simulink model "lab"  (Simulink 7.4)
settings: Solver=ode45  StartTime=0.0  StopTime=1  RelTol=1e-6
settings Model: Creator=im42741  LastModifiedBy=ks44349
settings OptimizationCC: InitFltsAndDblsToZero=on
settings DebuggingCC: SaveWithParameterizedLinksMsg=none  SignalResolutionControl=TryResolveAllWithWarning
settings GRTTargetCC: TargetFcnLib=ansi_tfl_tmw.mat

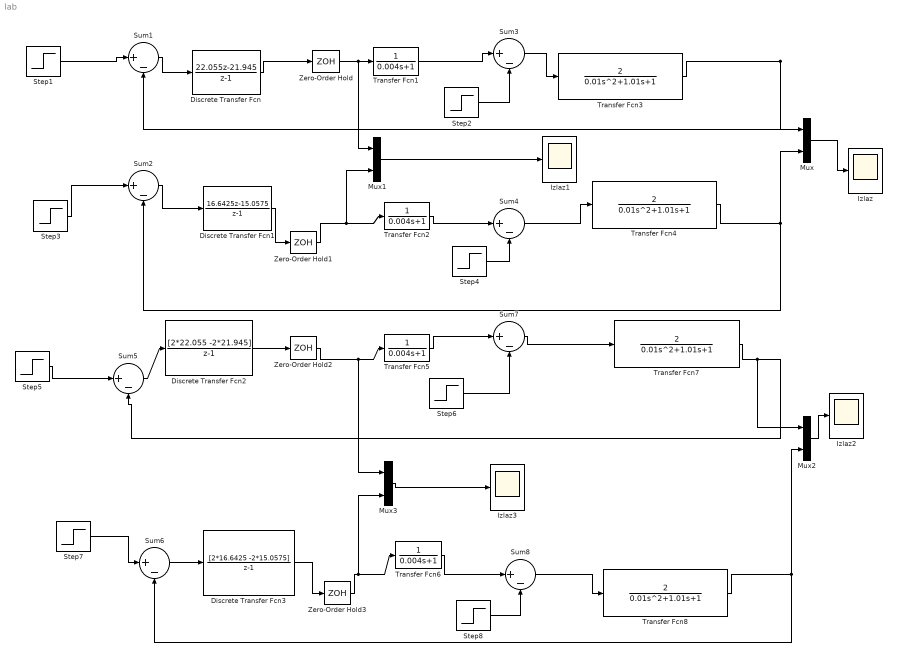
== system lab ==
  Discrete Transfer Fcn : DiscreteTransferFcn  Numerator=[22.055 -21.945]  Denominator=[1 -1]  SampleTime=5e-3
  Discrete Transfer Fcn1 : DiscreteTransferFcn  Numerator=[16.6425 -15.0575]  Denominator=[1 -1]  SampleTime=10e-3
  Discrete Transfer Fcn2 : DiscreteTransferFcn  Numerator=[2*22.055 -2*21.945]  Denominator=[1 -1]  SampleTime=0.004
  Discrete Transfer Fcn3 : DiscreteTransferFcn  Numerator=[2*16.6425 -2*15.0575]  Denominator=[1 -1]  SampleTime=0.004
  Izlaz{,1..3} (4 alike) : Scope
      Izlaz2 settings: SaveName=ScopeData2
      Izlaz3 settings: SaveName=ScopeData3
  Mux{,1..3} (4 alike) : Mux  Inputs=2
  Step{1,3,5,7} (4 alike) : Step  Time=0  After=0.1  SampleTime=0
  Step2 : Step  Time=0.5  SampleTime=0
  Step4 : Step  Time=0.05  SampleTime=0
  Step6 : Step  Time=0.05  SampleTime=0
  Step8 : Step  Time=0.05  SampleTime=0
  Sum{1..8} (8 alike) : Sum  Inputs=|+-  OutDataType=sfix(16)  OutScaling=2^0
  Transfer Fcn{1..2,5..6} (4 alike) : TransferFcn  Numerator=1  Denominator=[0.004 1]
  Transfer Fcn{3..4,7..8} (4 alike) : TransferFcn  Numerator=2  Denominator=[0.01 1.01 1]
  Zero-Order Hold : ZeroOrderHold  SampleTime=5e-3
  Zero-Order Hold1 : ZeroOrderHold  SampleTime=10e-3
  Zero-Order Hold2 : ZeroOrderHold  SampleTime=0.004
  Zero-Order Hold3 : ZeroOrderHold  SampleTime=0.004
  wires:
  Sum1/1 -> Discrete Transfer Fcn/1
  Transfer Fcn3/1 -> Sum1/2, Mux/1
  Discrete Transfer Fcn/1 -> Zero-Order Hold/1
  Mux/1 -> Izlaz/1
  Step1/1 -> Sum1/1
  Zero-Order Hold/1 -> Transfer Fcn1/1, Mux1/1
  Sum3/1 -> Transfer Fcn3/1
  Step2/1 -> Sum3/2
  Transfer Fcn1/1 -> Sum3/1
  Sum2/1 -> Discrete Transfer Fcn1/1
  Transfer Fcn4/1 -> Sum2/2, Mux/2
  Discrete Transfer Fcn1/1 -> Zero-Order Hold1/1
  Step3/1 -> Sum2/1
  Zero-Order Hold1/1 -> Transfer Fcn2/1, Mux1/2
  Sum4/1 -> Transfer Fcn4/1
  Step4/1 -> Sum4/2
  Transfer Fcn2/1 -> Sum4/1
  Mux1/1 -> Izlaz1/1
  Sum5/1 -> Discrete Transfer Fcn2/1
  Transfer Fcn7/1 -> Sum5/2, Mux2/1
  Discrete Transfer Fcn2/1 -> Zero-Order Hold2/1
  Mux2/1 -> Izlaz2/1
  Step5/1 -> Sum5/1
  Zero-Order Hold2/1 -> Transfer Fcn5/1, Mux3/1
  Sum7/1 -> Transfer Fcn7/1
  Step6/1 -> Sum7/2
  Transfer Fcn5/1 -> Sum7/1
  Sum6/1 -> Discrete Transfer Fcn3/1
  Transfer Fcn8/1 -> Sum6/2, Mux2/2
  Discrete Transfer Fcn3/1 -> Zero-Order Hold3/1
  Step7/1 -> Sum6/1
  Zero-Order Hold3/1 -> Transfer Fcn6/1, Mux3/2
  Sum8/1 -> Transfer Fcn8/1
  Step8/1 -> Sum8/2
  Transfer Fcn6/1 -> Sum8/1
  Mux3/1 -> Izlaz3/1
